simulink model "Mother_FIlter"  (R2019b)
settings: Solver=VariableStepAuto  StartTime=0.0  StopTime=5  MaxStep=1/100/pi/50  RelTol=1e-3
undefined symbols (not defined in the file or in its folder): wc
settings Model: Creator=mehdi  LastModifiedBy=mehdi

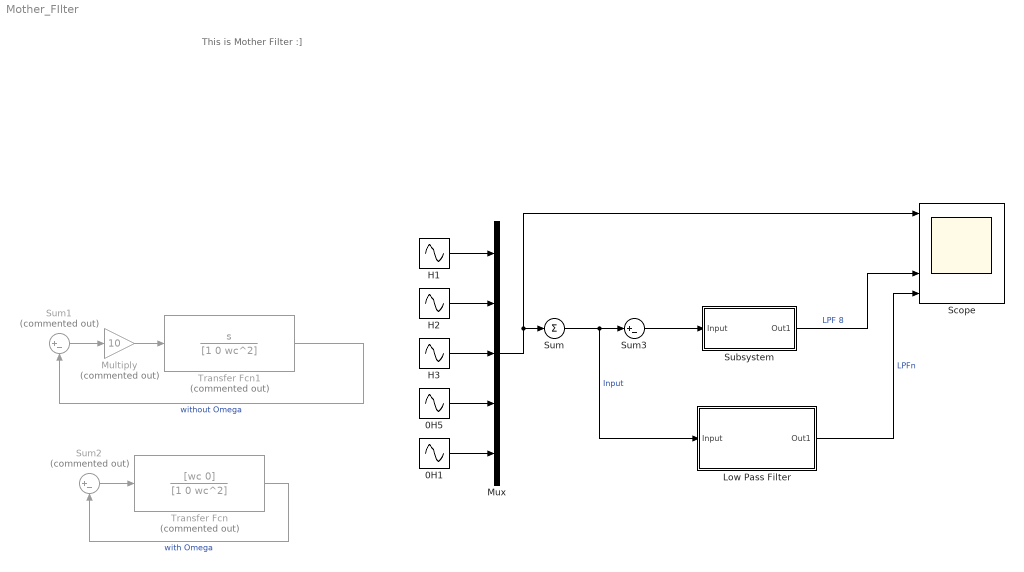
== system Mother_FIlter ==
  note: This is Mother Filter :]
  0H1 : Sin  Amplitude=20  Frequency=wc*0.1  SampleTime=0
  0H5 : Sin  Amplitude=20  Frequency=wc*0.5  SampleTime=0
  H1 : Sin  Amplitude=20  Frequency=wc  SampleTime=0
  H2 : Sin  Amplitude=20  Frequency=wc*2  SampleTime=0
  H3 : Sin  Amplitude=20  Frequency=wc*3  SampleTime=0
  Low Pass Filter : Subsystem  mask{f=1/2/pi, order=8, filter_num=[38865023.0418], filter_den=[1      50.265482457      1105.3956929      13890.811953      109098.18196 548387.27514      1722809.4349      3092780.2652      2429063.9401]}
      mask prompts: f "Cuttoff Freqeuncy"; order "Filter Order"; filter_num "Num"; filter_den "Den"
      mask DialogControl Designer Prompt: Designer
      mask DialogControl Designer Callback:
      | order = str2num(get_param(gcb, 'order'));
      | f = str2num(get_param(gcb, 'f'));
      | 
      | w = 2*pi*f;
      | 
      | den = [1];
      | for n=1:order
      |   den = conv(den, [1 w]);
      | end
      | 
      | filter = @(s) ( (w) / (s + w) )^order;
      | amp = abs( filter(1i*w) );
      | gain = 1 / amp;
      | g2 = gain;
      | disp([gain amp g2])
      | num = (w ^ order) * g2;
      | set_param(gcb, 'filter_num', strjoin({'[', num2str(num), ']'}, ''));
      | set_param(gcb, 'filter_den', strjoin({'[', num2str(den), ']'}, ''));
      mask Display: disp('Low Pass Filter')
  Multiply : Gain  Commented=on  Gain=10
  Mux : Mux  Inputs=5
  Scope : Scope  NumInputPorts=5
  Subsystem : Subsystem  mask{wc=1, g=16}
      mask prompts: wc "Cut-off Freqeuncy"; g "Gain"
      mask Display: disp('Low Pass Filter')
  Sum : Sum  Inputs=+
  Sum1 : Sum  Commented=on  Inputs=|+-
  Sum2 : Sum  Commented=on  Inputs=|+-
  Sum3 : Sum  Inputs=|+-
  Transfer Fcn : TransferFcn  Commented=on  Numerator=[wc 0]  Denominator=[1 0 wc^2]
  Transfer Fcn1 : TransferFcn  Commented=on  Numerator=[1 0]  Denominator=[1 0 wc^2]
  wires:
  Mux/1 -> Scope/1, Sum/1
  H1/1 -> Mux/1
  0H5/1 -> Mux/4
  H2/1 -> Mux/2
  H3/1 -> Mux/3
  Sum2/1 -> Transfer Fcn/1
  0H1/1 -> Mux/5
  Transfer Fcn/1 -> Sum2/2  "with Omega"
  Multiply/1 -> Transfer Fcn1/1
  Sum1/1 -> Multiply/1
  Transfer Fcn1/1 -> Sum1/2  "without Omega"
  Subsystem/1(Out1) -> Scope/4  "LPF 8"
  Sum3/1 -> Subsystem/1(Input)
  Sum/1 -> Low Pass Filter/1(Input), Sum3/1  "Input"
  Low Pass Filter/1(Out1) -> Scope/5  "LPFn"

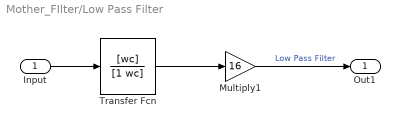
== system Mother_FIlter/Low Pass Filter ==
  Input : Inport
  Multiply1 : Gain  Gain=16
  Transfer Fcn : TransferFcn  Numerator=[wc]  Denominator=[1 wc]
  Out1 : Outport
  wires:
  Multiply1/1 -> Out1/1  "Low Pass Filter"
  Input/1 -> Transfer Fcn/1
  Transfer Fcn/1 -> Multiply1/1

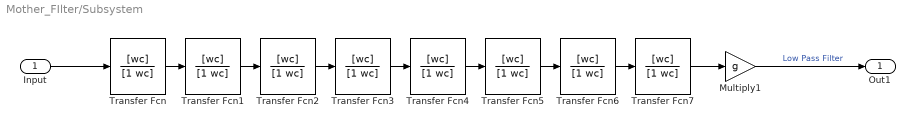
== system Mother_FIlter/Subsystem ==
  Input : Inport
  Multiply1 : Gain  Gain=g
  Transfer Fcn{,1..7} (8 alike) : TransferFcn  Numerator=[wc]  Denominator=[1 wc]
  Out1 : Outport
  wires:
  Transfer Fcn7/1 -> Multiply1/1
  Transfer Fcn6/1 -> Transfer Fcn7/1
  Transfer Fcn5/1 -> Transfer Fcn6/1
  Transfer Fcn2/1 -> Transfer Fcn3/1
  Transfer Fcn/1 -> Transfer Fcn1/1
  Transfer Fcn1/1 -> Transfer Fcn2/1
  Transfer Fcn4/1 -> Transfer Fcn5/1
  Input/1 -> Transfer Fcn/1
  Transfer Fcn3/1 -> Transfer Fcn4/1
  Multiply1/1 -> Out1/1  "Low Pass Filter"
